simulink model "test1_v4"  (R2018a)
settings: Solver=VariableStepAuto  StartTime=0.0  StopTime=100  FixedStep=0.01  RelTol=1e-3  EnableMultiTasking=on
InitFcn:
  | run constants
values from neighbouring files (symbols this model uses):
  F_0 = [0 0 0]    [constants2.m]
  phi_noise = noise_att_on * noise_att_mag    [constants2.m]
  pm_0 = [0 0 0]    [constants2.m]
  Psi_noise = noise_att_on * noise_att_mag    [constants2.m]
  R = (RE + 700*1000)    (= 7078000)    [constants2.m]
  T_d = Td_on * [0.001 0.001 0.001]    [constants2.m]
  theta_noise = noise_att_on * noise_att_mag    [constants2.m]
  Vm_0 = [0 Vc 0]    [constants2.m]
  xme_0 = [1 2 3]    [constants2.m]
undefined symbols (not defined in the file or in its folder): Discrete, n, phi_D, phi_I, phi_P, pqr_noise, Psi_D, Psi_I, Psi_P, theta_D, theta_I, theta_P, Time
libraries: shared6dof x5, simulink x4, shared6dofsys x3, sharedutil x1, sharedTrackingLibrary x1, ctrlSharedLib x1
settings Model: PacingRate=1000  Creator=Matt  LastModifiedBy=matth
settings SolverCC: AutoInsertRateTranBlk=on
settings DataIOCC: SaveOutput=off  SaveTime=off
settings OptimizationCC: DefaultParameterBehavior=Inlined  InlineInvariantSignals=on  EnhancedBackFolding=on  PassReuseOutputArgsAs=Individual arguments  StateBitsets=on  DataBitsets=on  ZeroExternalMemoryAtStartup=off  ZeroInternalMemoryAtStartup=off  NoFixptDivByZeroProtection=on  LifeSpan=1  OptimizeBlockOrder=speed  DifferentSizesBufferReuse=on
settings DebuggingCC: ParameterTunabilityLossMsg=error
settings HardwareCC: ProdBitPerPointer=32  ProdBitPerSizeT=32  ProdBitPerPtrDiffT=32  ProdLargestAtomicFloat=None  ProdIntDivRoundTo=Floor  ProdWordSize=32  ProdHWDeviceType=Generic->Custom
settings SFSimCC: MATLABDynamicMemAlloc=off
settings RTWCC: SystemTargetFile=ert.tlc  TLCOptions=-p0  GenCodeOnly=on  TemplateMakefile=ert_default_tmf  GenerateReport=on  RTWVerbose=off  IncludeHyperlinkInReport=on  LaunchReport=on  GenerateTraceInfo=on  GenerateTraceReport=on  GenerateTraceReportSl=on  GenerateTraceReportSf=on  GenerateTraceReportEml=on
settings CodeAppCC: ForceParamTrailComments=on  IgnoreCustomStorageClasses=off  OperatorAnnotations=on  SimulinkDataObjDesc=on  SFDataObjDesc=on  CustomSymbolStrGlobalVar=rt$N$M  CustomSymbolStrType=$N$M  CustomSymbolStrFcn=$N$M$F  CustomSymbolStrMacro=$N$M  InsertBlockDesc=on
settings ERTTargetCC: TargetLangStandard=C99 (ISO)  CodeReplacementLibrary=ISO_C  GenerateSampleERTMain=on  IncludeMdlTerminateFcn=off  SuppressErrorStatus=on  SupportAbsoluteTime=off  SupportNonFinite=off  SupportComplex=off  PurelyIntegerCode=on  InlinedParameterPlacement=NonHierarchical  RootIOFormat=Structure reference  ERTCustomFileTemplate=example_file_process.tlc

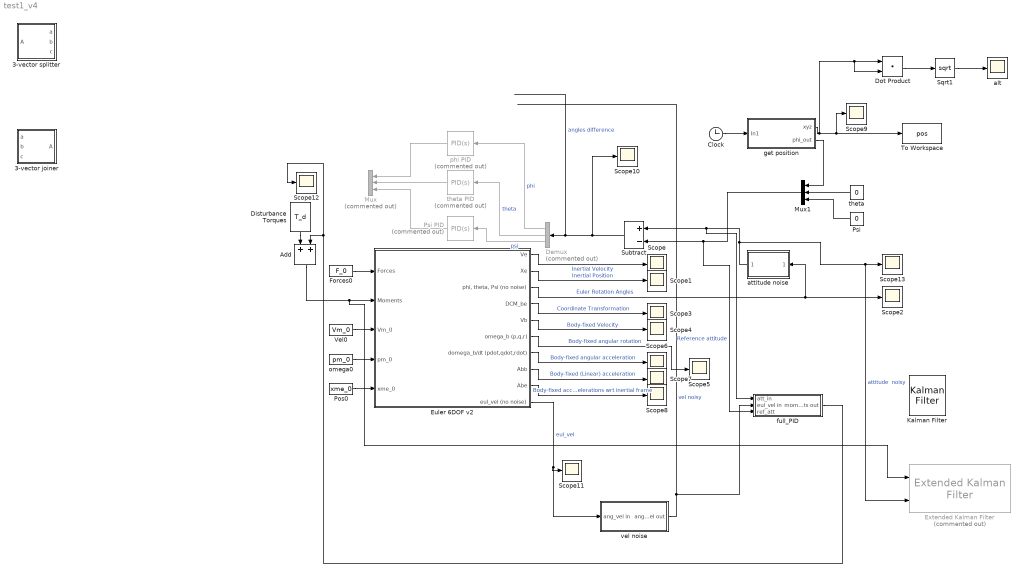
== system test1_v4 ==
  3-vector joiner : Subsystem
  3-vector splitter : Subsystem
  Add : Sum
  Clock : Clock
  Demux : Demux  Commented=on  Outputs=3
  Disturbance Torques : Constant  Value=T_d
  Dot Product : DotProduct  InputSameDT=on  OutDataTypeStr=Inherit: Inherit via internal rule
  Euler 6DOF v2 : Subsystem
  Extended Kalman Filter : sharedTrackingLibrary/Extended Kalman Filter  Commented=on  StateTransitionFcn=myStateTransitionFcn  HasStateTransitionJacobianFcn=off  HasAdditiveProcessNoise=Additive  ProcessNoise=1  HasTimeVaryingProcessNoise=off  HasStateTransitionFcnExtraArgument=1  InitialState=0  InitialStateCovariance=1  MeasurementFcn1=myMeasurementFcn  HasMeasurementJacobianFcn1=off  HasMeasurementEnablePort1=off  HasAdditiveMeasurementNoise1=Additive  MeasurementNoise1=1  HasTimeVaryingMeasurementNoise1=off  HasMeasurementFcnExtraArgument1=0  MeasurementFcn2=myMeasurementFcn  HasMeasurementJacobianFcn2=off  HasMeasurementEnablePort2=off  HasAdditiveMeasurementNoise2=Additive  MeasurementNoise2=1  HasTimeVaryingMeasurementNoise2=off  HasMeasurementFcnExtraArgument2=0  MeasurementFcn3=myMeasurementFcn  HasMeasurementJacobianFcn3=off  HasMeasurementEnablePort3=off  HasAdditiveMeasurementNoise3=Additive  MeasurementNoise3=1  HasTimeVaryingMeasurementNoise3=off  HasMeasurementFcnExtraArgument3=0  MeasurementFcn4=myMeasurementFcn  HasMeasurementJacobianFcn4=off  HasMeasurementEnablePort4=off  HasAdditiveMeasurementNoise4=Additive  MeasurementNoise4=1  HasTimeVaryingMeasurementNoise4=off  HasMeasurementFcnExtraArgument4=0  MeasurementFcn5=myMeasurementFcn  HasMeasurementJacobianFcn5=off  HasMeasurementEnablePort5=off  HasAdditiveMeasurementNoise5=Additive  MeasurementNoise5=1  HasTimeVaryingMeasurementNoise5=off  HasMeasurementFcnExtraArgument5=0  EnableMultirate=off  StateTransitionFcnSampleTime=1  MeasurementFcn1SampleTime=1  MeasurementFcn2SampleTime=1  MeasurementFcn3SampleTime=1  MeasurementFcn4SampleTime=1  MeasurementFcn5SampleTime=1  UseCurrentEstimator=off  OutputStateCovariance=off  DataType=double  SampleTime=1  NumberOfMeasurements=1
      settings: SourceProductName=Control System Toolbox  SourceProductBaseCode=CT
  Forces0 : Constant  Value=F_0
  Kalman Filter : ctrlSharedLib/Kalman Filter  TimeDomain=Discrete-Time  UseCurrentEstimator=on  ModelSource=LTI State-Space Variable  ModelSourceVariable=ss(0.95,1,1,0,1)  A=0.95  B=1  C=1  D=0  NumberOfStates=1  NumberOfInputs=1  NumberOfOutputs=1  InitialEstimateSource=Dialog  X0=0  P0=10  UseK=off  UseGH=off  NumberOfProcessNoiseInputs=1  G=1  TimeInvariantG=on  H=0  TimeInvariantH=on  Q=0.05  TimeInvariantQ=on  R=1  TimeInvariantR=on  N=0  TimeInvariantN=on  AddInputPort=on  AddEnablePort=off  OutputEstimatedY=off  OutputP=off  Ts=-1
      settings: SourceProductBaseCode=CT
  Mux : Mux  Commented=on  Inputs=3
  Mux1 : Mux  Inputs=3
  Pos0 : Constant  Value=xme_0
  "Psi " : Constant  Value=0
  Psi PID : simulink/Continuous/PID Controller  Commented=on  Controller=PID  TimeDomain=Continuous-time  SampleTime=-1  IntegratorMethod=Forward Euler  FilterMethod=Forward Euler  Form=Parallel  UseFilter=on  ControllerParametersSource=internal  P=-7886.12074600839  I=-460.070676690981  D=-30034.6975048403  N=1142.8279760416  InitialConditionSource=internal  InitialConditionForIntegrator=0  InitialConditionForFilter=0  ExternalReset=none  LimitOutput=off  UpperSaturationLimit=inf  LowerSaturationLimit=-inf  LinearizeAsGain=on  AntiWindupMode=none  Kb=1  TrackingMode=off  Kt=1  PParamMin=[]  PParamMax=[]  IParamMin=[]  IParamMax=[]  DParamMin=[]  DParamMax=[]  NParamMin=[]  NParamMax=[]  KbParamMin=[]  KbParamMax=[]  KtParamMin=[]  KtParamMax=[]  POutMin=[]  POutMax=[]  IOutMin=[]  IOutMax=[]  DOutMin=[]  DOutMax=[]  NOutMin=[]  NOutMax=[]  KbOutMin=[]  KbOutMax=[]  KtOutMin=[]  KtOutMax=[]  IntegratorOutMin=[]  IntegratorOutMax=[]  FilterOutMin=[]  FilterOutMax=[]  SumOutMin=[]  SumOutMax=[]  SumI1OutMin=[]  SumI1OutMax=[]  SumI2OutMin=[]  SumI2OutMax=[]  SumI3OutMin=[]  SumI3OutMax=[]  SumDOutMin=[]  SumDOutMax=[]  SaturationOutMin=[]  SaturationOutMax=[]  IntegratorContinuousStateAttributes=''  IntegratorStateMustResolveToSignalObject=off  IntegratorRTWStateStorageClass=Auto  FilterContinuousStateAttributes=''  FilterStateMustResolveToSignalObject=off  FilterRTWStateStorageClass=Auto  DifferentiatorICPrevScaledInput=0  DifferentiatorOutMin=[]  DifferentiatorOutMax=[]  FilterDiffOutCoefMin=[]  FilterDiffOutCoefMax=[]  SumDenOutMin=[]  SumDenOutMax=[]  SumNumOutMin=[]  SumNumOutMax=[]  ReciprocalOutMin=[]  ReciprocalOutMax=[]  DivideOutMin=[]  DivideOutMax=[]  TunerSelectOption=Transfer Function Based (PID Tuner App)
  Scope{,1..13} (14 alike) : Scope
  Sqrt1 : Sqrt  SaturateOnIntegerOverflow=on
  Subtract : Sum  Inputs=+-
  To Workspace : ToWorkspace  VariableName=pos  SaveFormat=Timeseries  SampleTime=-1
  Vel0 : Constant  Value=Vm_0
  alt : Scope
  attitude noise : Subsystem
  "full_PID " : Subsystem
  get position : Subsystem
  "omega0 " : Constant  Value=pm_0
  "phi PID " : simulink/Continuous/PID Controller  Commented=on  Controller=PID  TimeDomain=Continuous-time  SampleTime=-1  IntegratorMethod=Forward Euler  FilterMethod=Forward Euler  Form=Parallel  UseFilter=on  ControllerParametersSource=internal  P=-464.198158177747  I=-21.7313338529705  D=-2434.80245399495  N=5.45397025421619  InitialConditionSource=internal  InitialConditionForIntegrator=0  InitialConditionForFilter=0  ExternalReset=none  LimitOutput=off  UpperSaturationLimit=inf  LowerSaturationLimit=-inf  LinearizeAsGain=on  AntiWindupMode=none  Kb=1  TrackingMode=off  Kt=1  PParamMin=[]  PParamMax=[]  IParamMin=[]  IParamMax=[]  DParamMin=[]  DParamMax=[]  NParamMin=[]  NParamMax=[]  KbParamMin=[]  KbParamMax=[]  KtParamMin=[]  KtParamMax=[]  POutMin=[]  POutMax=[]  IOutMin=[]  IOutMax=[]  DOutMin=[]  DOutMax=[]  NOutMin=[]  NOutMax=[]  KbOutMin=[]  KbOutMax=[]  KtOutMin=[]  KtOutMax=[]  IntegratorOutMin=[]  IntegratorOutMax=[]  FilterOutMin=[]  FilterOutMax=[]  SumOutMin=[]  SumOutMax=[]  SumI1OutMin=[]  SumI1OutMax=[]  SumI2OutMin=[]  SumI2OutMax=[]  SumI3OutMin=[]  SumI3OutMax=[]  SumDOutMin=[]  SumDOutMax=[]  SaturationOutMin=[]  SaturationOutMax=[]  IntegratorContinuousStateAttributes=''  IntegratorStateMustResolveToSignalObject=off  IntegratorRTWStateStorageClass=Auto  FilterContinuousStateAttributes=''  FilterStateMustResolveToSignalObject=off  FilterRTWStateStorageClass=Auto  DifferentiatorICPrevScaledInput=0  DifferentiatorOutMin=[]  DifferentiatorOutMax=[]  FilterDiffOutCoefMin=[]  FilterDiffOutCoefMax=[]  SumDenOutMin=[]  SumDenOutMax=[]  SumNumOutMin=[]  SumNumOutMax=[]  ReciprocalOutMin=[]  ReciprocalOutMax=[]  DivideOutMin=[]  DivideOutMax=[]  TunerSelectOption=Transfer Function Based (PID Tuner App)
  theta : Constant  Value=0
  theta PID : simulink/Continuous/PID Controller  Commented=on  Controller=PID  TimeDomain=Continuous-time  SampleTime=-1  IntegratorMethod=Forward Euler  FilterMethod=Forward Euler  Form=Parallel  UseFilter=on  ControllerParametersSource=internal  P=-568.423410964435  I=-28.5001924417647  D=-2213.03320065217  N=10.4897155810233  InitialConditionSource=internal  InitialConditionForIntegrator=0  InitialConditionForFilter=0  ExternalReset=none  LimitOutput=off  UpperSaturationLimit=inf  LowerSaturationLimit=-inf  LinearizeAsGain=on  AntiWindupMode=none  Kb=1  TrackingMode=off  Kt=1  PParamMin=[]  PParamMax=[]  IParamMin=[]  IParamMax=[]  DParamMin=[]  DParamMax=[]  NParamMin=[]  NParamMax=[]  KbParamMin=[]  KbParamMax=[]  KtParamMin=[]  KtParamMax=[]  POutMin=[]  POutMax=[]  IOutMin=[]  IOutMax=[]  DOutMin=[]  DOutMax=[]  NOutMin=[]  NOutMax=[]  KbOutMin=[]  KbOutMax=[]  KtOutMin=[]  KtOutMax=[]  IntegratorOutMin=[]  IntegratorOutMax=[]  FilterOutMin=[]  FilterOutMax=[]  SumOutMin=[]  SumOutMax=[]  SumI1OutMin=[]  SumI1OutMax=[]  SumI2OutMin=[]  SumI2OutMax=[]  SumI3OutMin=[]  SumI3OutMax=[]  SumDOutMin=[]  SumDOutMax=[]  SaturationOutMin=[]  SaturationOutMax=[]  IntegratorContinuousStateAttributes=''  IntegratorStateMustResolveToSignalObject=off  IntegratorRTWStateStorageClass=Auto  FilterContinuousStateAttributes=''  FilterStateMustResolveToSignalObject=off  FilterRTWStateStorageClass=Auto  DifferentiatorICPrevScaledInput=0  DifferentiatorOutMin=[]  DifferentiatorOutMax=[]  FilterDiffOutCoefMin=[]  FilterDiffOutCoefMax=[]  SumDenOutMin=[]  SumDenOutMax=[]  SumNumOutMin=[]  SumNumOutMax=[]  ReciprocalOutMin=[]  ReciprocalOutMax=[]  DivideOutMin=[]  DivideOutMax=[]  TunerSelectOption=Transfer Function Based (PID Tuner App)
  "vel noise " : Subsystem
  wires:
  Euler 6DOF v2/1(Ve) -> Scope/1  "Inertial Velocity"
  Euler 6DOF v2/2(Xe) -> Scope1/1  "Inertial Position"
  Euler 6DOF v2/3("phi, theta, Psi (no noise)") -> attitude noise/1(att_in), Scope2/1  "Euler Rotation Angles"
  Euler 6DOF v2/4(DCM_be) -> Scope3/1  "Coordinate Transformation"
  Euler 6DOF v2/5(Vb) -> Scope4/1  "Body-fixed Velocity"
  Euler 6DOF v2/6(omega_b (p,q,r)) -> Scope5/1  "Body-fixed angular rotation"
  Euler 6DOF v2/7(domega_b/dt (pdot,qdot,rdot)) -> Scope6/1  "Body-fixed angular acceleration"
  Euler 6DOF v2/8(Abb) -> Scope7/1  "Body-fixed (Linear) acceleration"
  Euler 6DOF v2/9(Abe) -> Scope8/1  "Body-fixed accelerations wrt inertial frame"
  Mux1/1 -> "full_PID "/3(ref_att), Subtract/2  "Reference attitude"
  Demux/1 -> "phi PID "/1  "phi"
  Demux/2 -> theta PID/1  "theta"
  Demux/3 -> Psi PID/1  "psi"
  "phi PID "/1 -> Mux/1
  theta PID/1 -> Mux/2
  Psi PID/1 -> Mux/3
  "full_PID "/1(moments out) -> Scope12/1, Add/2
  Subtract/1 -> Scope10/1, Demux/1  "angles difference"
  Forces0/1 -> Euler 6DOF v2/1(Forces)
  Vel0/1 -> Euler 6DOF v2/3(Vm_0)
  Pos0/1 -> Euler 6DOF v2/5("xme_0 ")
  "omega0 "/1 -> Euler 6DOF v2/4("pm_0 ")
  Disturbance Torques/1 -> Add/1
  Add/1 -> Extended Kalman Filter/1, Euler 6DOF v2/2(Moments)
  Dot Product/1 -> Sqrt1/1
  Sqrt1/1 -> alt/1
  Clock/1 -> get position/1(In1)
  get position/1(xyz) -> Dot Product/2, Dot Product/1, To Workspace/1, Scope9/1
  Euler 6DOF v2/10(eul_vel (no noise)) -> "vel noise "/1(ang_vel in), Scope11/1  "eul_vel"
  attitude noise/1("att_out ") -> "full_PID "/1(att_in), Subtract/1, Extended Kalman Filter/2, Scope13/1  "attitude  noisy"
  "vel noise "/1(ang_vel out) -> "full_PID "/2(eul_vel in)  "vel noisy"
  get position/2(phi_out) -> Mux1/1
  "Psi "/1 -> Mux1/3
  theta/1 -> Mux1/2

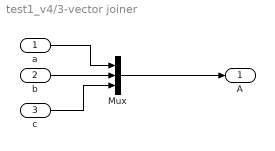
== system test1_v4/3-vector joiner ==
  a : Inport
  b : Inport  Port=2
  c : Inport  Port=3
  Mux : Mux  Inputs=3
  A : Outport
  wires:
  c/1 -> Mux/3
  a/1 -> Mux/1
  b/1 -> Mux/2
  Mux/1 -> A/1

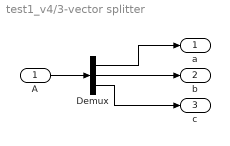
== system test1_v4/3-vector splitter ==
  A : Inport
  Demux : Demux  Outputs=3
  a : Outport
  b : Outport  Port=2
  c : Outport  Port=3
  wires:
  Demux/3 -> c/1
  Demux/2 -> b/1
  Demux/1 -> a/1
  A/1 -> Demux/1

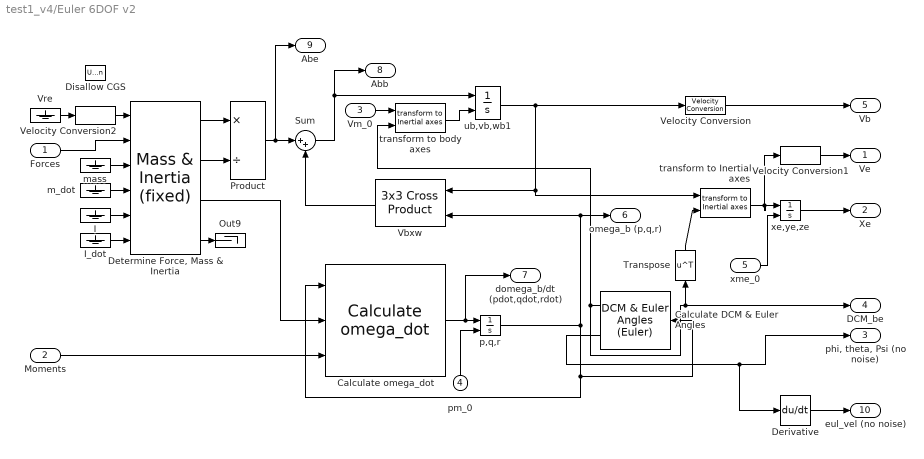
== system test1_v4/Euler 6DOF v2 ==
  Forces : Inport  Unit=N  PortDimensions=3
  Moments : Inport  Port=2  Unit=N*m  PortDimensions=3
  Vm_0 : Inport  Port=3
  "pm_0 " : Inport  Port=4
  "xme_0 " : Inport  Port=5
  Calculate DCM & Euler Angles : shared6dofsys/DCM & Euler Angles (Euler)  aMode=aMode
      settings: SourceProductName=Aerospace Blockset  SourceProductBaseCode=AE
  Calculate omega_dot : shared6dofsys/Calculate omega_dot  aMode=aMode
      settings: SourceProductName=Aerospace Blockset  SourceProductBaseCode=AE
  Derivative : Derivative
  "Determine Force, Mass & Inertia" : shared6dofsys/Mass & Inertia (fixed)  aMode=aMode
      settings: SourceProductName=Aerospace Blockset  SourceProductBaseCode=AE
  Disallow CGS : UnitConfiguration  UnitSystemsStr=English,SI,SI (extended)  AllowAllUnitSystems=off
  I : Ground
  I_dot : Ground
  Out9 : Terminator
  Product : Product  Inputs=*/  SaturateOnIntegerOverflow=on  OutDataTypeStr=Inherit: Same as first input
  Sum : Sum  Inputs=|++  SaturateOnIntegerOverflow=on
  Transpose : Math  Operator=transpose  SaturateOnIntegerOverflow=on
  Vbxw : sharedutil/3x3 Cross Product  aMode=aMode
      settings: SourceProductBaseCode=AE
  Velocity Conversion : shared6dof/6DOF (Euler Angles)/Velocity Conversion
      settings: SourceProductName=Aerospace Blockset  SourceProductBaseCode=AE
  Velocity Conversion1 : shared6dof/6DOF (Euler Angles)/Velocity Conversion1
      settings: SourceProductName=Aerospace Blockset  SourceProductBaseCode=AE
  Velocity Conversion2 : shared6dof/6DOF (Euler Angles)/Velocity Conversion2
      settings: SourceProductName=Aerospace Blockset  SourceProductBaseCode=AE
  Vre : Ground
  m_dot : Ground
  mass : Ground
  "p,q,r " : Integrator  InitialConditionSource=external  InitialCondition=pm_0
  "transform to Inertial axes " : shared6dof/6DOF (Euler Angles)/transform to Inertial axes   SystemSampleTime=-1
      settings: SourceProductName=Aerospace Blockset  SourceProductBaseCode=AE
  transform to body axes : shared6dof/6DOF (Euler Angles)/transform to Inertial axes   SystemSampleTime=-1
      settings: SourceProductName=Aerospace Blockset  SourceProductBaseCode=AE
  ub,vb,wb1 : Integrator  InitialConditionSource=external  InitialCondition=Vm_0
  xe,ye,ze : Integrator  InitialConditionSource=external  InitialCondition=xme_0
  Ve : Outport  Unit=m/s
  Xe : Outport  Port=2  Unit=m
  "phi, theta, Psi (no noise)" : Outport  Port=3  Unit=rad
  DCM_be : Outport  Port=4  Unit=1
  Vb : Outport  Port=5  Unit=m/s
  omega_b (p,q,r) : Outport  Port=6  Unit=rad/s
  domega_b/dt (pdot,qdot,rdot) : Outport  Port=7  Unit=rad/s^2
  Abb : Outport  Port=8  Unit=m/s^2
  Abe : Outport  Port=9  Unit=m/s^2
  eul_vel (no noise) : Outport  Port=10
  wires:
  Calculate DCM & Euler Angles/1 -> transform to body axes/2, Transpose/1, DCM_be/1
  Vbxw/1 -> Sum/2
  Velocity Conversion/1 -> Vb/1
  xe,ye,ze/1 -> Xe/1
  Vre/1 -> Velocity Conversion2/1
  Calculate DCM & Euler Angles/2 -> Derivative/1, "phi, theta, Psi (no noise)"/1
  "p,q,r "/1 -> Calculate omega_dot/1, Calculate DCM & Euler Angles/1, omega_b (p,q,r)/1, Vbxw/2
  Product/1 -> Sum/1, Abe/1
  Moments/1 -> Calculate omega_dot/3
  "Determine Force, Mass & Inertia"/2 -> Product/2
  "transform to Inertial axes "/1 -> xe,ye,ze/1, Velocity Conversion1/1
  "Determine Force, Mass & Inertia"/4 -> Out9/1
  Transpose/1 -> "transform to Inertial axes "/2
  mass/1 -> "Determine Force, Mass & Inertia"/3
  Velocity Conversion1/1 -> Ve/1
  Calculate omega_dot/1 -> "p,q,r "/1, domega_b/dt (pdot,qdot,rdot)/1
  I/1 -> "Determine Force, Mass & Inertia"/5
  "Determine Force, Mass & Inertia"/3 -> Calculate omega_dot/2
  ub,vb,wb1/1 -> "transform to Inertial axes "/1, Vbxw/1, Velocity Conversion/1
  "Determine Force, Mass & Inertia"/1 -> Product/1
  Forces/1 -> "Determine Force, Mass & Inertia"/2
  Velocity Conversion2/1 -> "Determine Force, Mass & Inertia"/1
  I_dot/1 -> "Determine Force, Mass & Inertia"/6
  Sum/1 -> Abb/1, ub,vb,wb1/1
  m_dot/1 -> "Determine Force, Mass & Inertia"/4
  Vm_0/1 -> transform to body axes/1
  "pm_0 "/1 -> "p,q,r "/2
  "xme_0 "/1 -> xe,ye,ze/2
  transform to body axes/1 -> ub,vb,wb1/2
  Derivative/1 -> eul_vel (no noise)/1

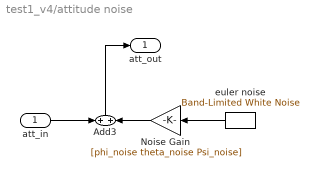
== system test1_v4/attitude noise ==
  att_in : Inport
  Add3 : Sum
  Noise Gain : Gain  Gain=[phi_noise theta_noise Psi_noise]
  euler noise : simulink/Sources/Band-Limited White Noise  Cov=[0.1]  Ts=0.1  seed=[23341]
  "att_out " : Outport
  wires:
  euler noise/1 -> Noise Gain/1
  Noise Gain/1 -> Add3/2
  att_in/1 -> Add3/1
  Add3/1 -> "att_out "/1

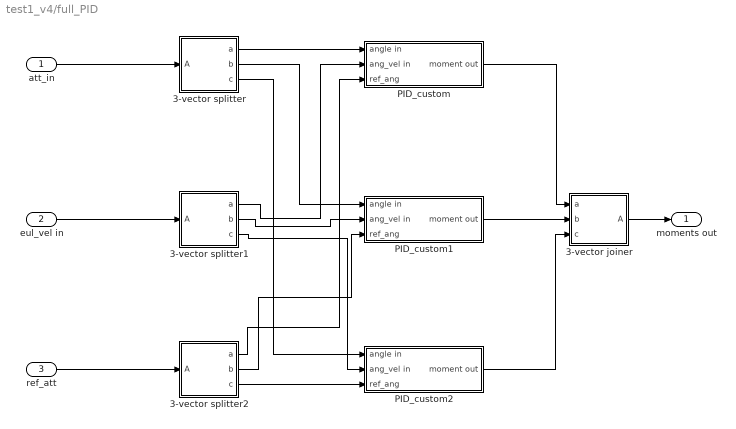
== system test1_v4/full_PID  ==
  att_in : Inport
  eul_vel in : Inport  Port=2
  ref_att : Inport  Port=3
  3-vector joiner : Subsystem
  3-vector splitter : Subsystem
  3-vector splitter1 : Subsystem
  3-vector splitter2 : Subsystem
  PID_custom : Subsystem
  PID_custom1 : Subsystem
  PID_custom2 : Subsystem
  moments out : Outport  InitialOutput=0
  wires:
  att_in/1 -> 3-vector splitter/1(A)
  eul_vel in/1 -> 3-vector splitter1/1(A)
  ref_att/1 -> 3-vector splitter2/1(A)
  3-vector splitter/1(a) -> PID_custom/1(angle in)
  3-vector splitter/2(b) -> PID_custom1/1(angle in)
  3-vector splitter/3(c) -> PID_custom2/1(angle in)
  3-vector splitter1/1(a) -> PID_custom/2(ang_vel in)
  3-vector splitter1/2(b) -> PID_custom1/2(ang_vel in)
  3-vector splitter1/3(c) -> PID_custom2/2(ang_vel in)
  3-vector splitter2/1(a) -> PID_custom/3("ref_ang ")
  3-vector splitter2/2(b) -> PID_custom1/3("ref_ang ")
  3-vector splitter2/3(c) -> PID_custom2/3("ref_ang ")
  PID_custom1/1("moment out ") -> 3-vector joiner/2(b)
  PID_custom/1("moment out ") -> 3-vector joiner/1(a)
  PID_custom2/1("moment out ") -> 3-vector joiner/3(c)
  3-vector joiner/1(A) -> moments out/1

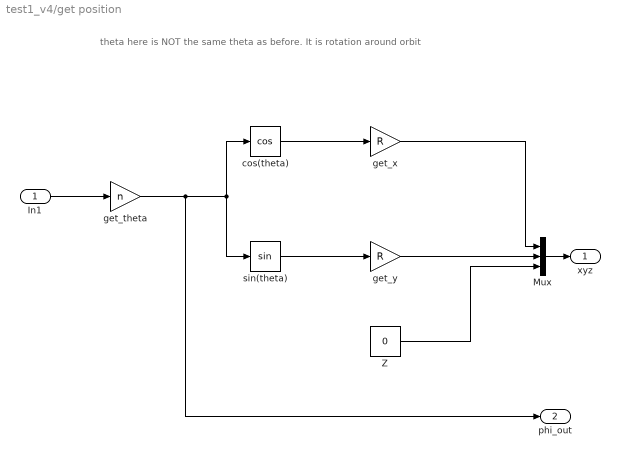
== system test1_v4/get position ==
  note: theta here is NOT the same theta as before. It is rotation around orbit
  In1 : Inport
  Mux : Mux  Inputs=3
  "Z " : Constant  Value=0
  cos(theta) : Trigonometry  Operator=cos
  get_theta : Gain  Gain=n
  "get_x " : Gain  Gain=R
  get_y : Gain  Gain=R
  sin(theta) : Trigonometry
  xyz : Outport
  phi_out : Outport  Port=2
  wires:
  In1/1 -> get_theta/1
  get_theta/1 -> phi_out/1, cos(theta)/1, sin(theta)/1
  cos(theta)/1 -> "get_x "/1
  sin(theta)/1 -> get_y/1
  "Z "/1 -> Mux/3
  get_y/1 -> Mux/2
  "get_x "/1 -> Mux/1
  Mux/1 -> xyz/1

== system test1_v4/vel noise  ==
  ang_vel in : Inport
  Add : Sum
  pqr_noise : Constant  Value=pqr_noise
  ang_vel out : Outport
  wires:
  ang_vel in/1 -> Add/2
  pqr_noise/1 -> Add/1
  Add/1 -> ang_vel out/1

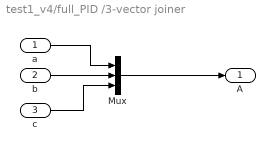
== system test1_v4/full_PID /3-vector joiner ==
  a : Inport
  b : Inport  Port=2
  c : Inport  Port=3
  Mux : Mux  Inputs=3
  A : Outport
  wires:
  c/1 -> Mux/3
  a/1 -> Mux/1
  b/1 -> Mux/2
  Mux/1 -> A/1

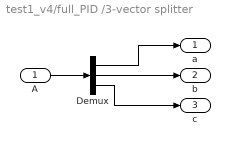
== system test1_v4/full_PID /3-vector splitter ==
  A : Inport
  Demux : Demux  Outputs=3
  a : Outport
  b : Outport  Port=2
  c : Outport  Port=3
  wires:
  Demux/3 -> c/1
  Demux/2 -> b/1
  Demux/1 -> a/1
  A/1 -> Demux/1

== system test1_v4/full_PID /3-vector splitter1 ==
  A : Inport
  Demux : Demux  Outputs=3
  a : Outport
  b : Outport  Port=2
  c : Outport  Port=3
  wires:
  Demux/3 -> c/1
  Demux/2 -> b/1
  Demux/1 -> a/1
  A/1 -> Demux/1

== system test1_v4/full_PID /3-vector splitter2 ==
  A : Inport
  Demux : Demux  Outputs=3
  a : Outport
  b : Outport  Port=2
  c : Outport  Port=3
  wires:
  Demux/3 -> c/1
  Demux/2 -> b/1
  Demux/1 -> a/1
  A/1 -> Demux/1

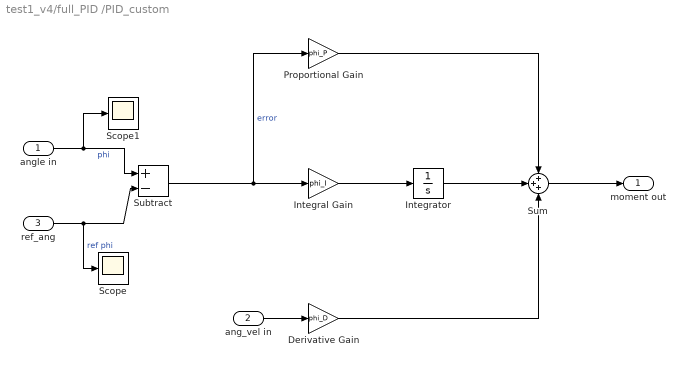
== system test1_v4/full_PID /PID_custom ==
  angle in : Inport
  ang_vel in : Inport  Port=2
  "ref_ang " : Inport  Port=3
  Derivative Gain : Gain  Gain=phi_D
  Integral Gain : Gain  Gain=phi_I
  Integrator : Integrator
  Proportional Gain : Gain  Gain=phi_P
  Scope : Scope
  Scope1 : Scope
  Subtract : Sum  Inputs=+-
  Sum : Sum  Inputs=+++
  "moment out " : Outport
  wires:
  angle in/1 -> Scope1/1, Subtract/1  "phi"
  "ref_ang "/1 -> Scope/1, Subtract/2  "ref phi"
  Subtract/1 -> Integral Gain/1, Proportional Gain/1  "error"
  Integral Gain/1 -> Integrator/1
  Proportional Gain/1 -> Sum/1
  Integrator/1 -> Sum/2
  ang_vel in/1 -> Derivative Gain/1
  Derivative Gain/1 -> Sum/3
  Sum/1 -> "moment out "/1

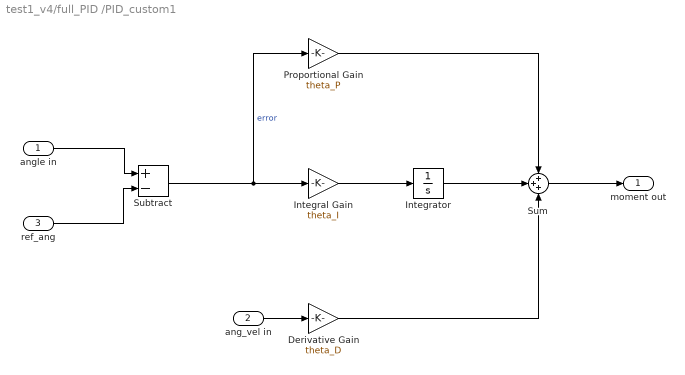
== system test1_v4/full_PID /PID_custom1 ==
  angle in : Inport
  ang_vel in : Inport  Port=2
  "ref_ang " : Inport  Port=3
  Derivative Gain : Gain  Gain=theta_D
  Integral Gain : Gain  Gain=theta_I
  Integrator : Integrator
  Proportional Gain : Gain  Gain=theta_P
  Subtract : Sum  Inputs=+-
  Sum : Sum  Inputs=+++
  "moment out " : Outport
  wires:
  angle in/1 -> Subtract/1
  "ref_ang "/1 -> Subtract/2
  Subtract/1 -> Integral Gain/1, Proportional Gain/1  "error"
  Integral Gain/1 -> Integrator/1
  Proportional Gain/1 -> Sum/1
  Integrator/1 -> Sum/2
  ang_vel in/1 -> Derivative Gain/1
  Derivative Gain/1 -> Sum/3
  Sum/1 -> "moment out "/1

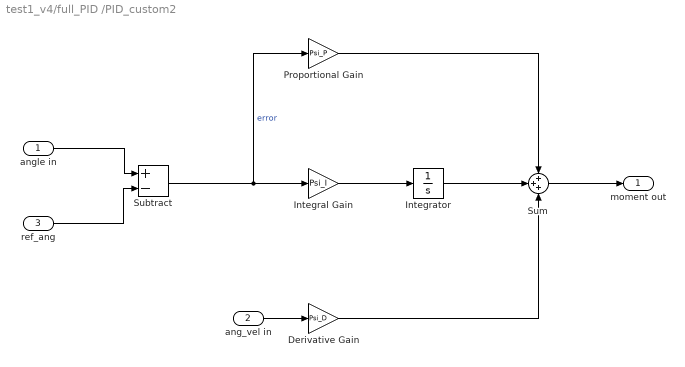
== system test1_v4/full_PID /PID_custom2 ==
  angle in : Inport
  ang_vel in : Inport  Port=2
  "ref_ang " : Inport  Port=3
  Derivative Gain : Gain  Gain=Psi_D
  Integral Gain : Gain  Gain=Psi_I
  Integrator : Integrator
  Proportional Gain : Gain  Gain=Psi_P
  Subtract : Sum  Inputs=+-
  Sum : Sum  Inputs=+++
  "moment out " : Outport
  wires:
  angle in/1 -> Subtract/1
  "ref_ang "/1 -> Subtract/2
  Subtract/1 -> Integral Gain/1, Proportional Gain/1  "error"
  Integral Gain/1 -> Integrator/1
  Proportional Gain/1 -> Sum/1
  Integrator/1 -> Sum/2
  ang_vel in/1 -> Derivative Gain/1
  Derivative Gain/1 -> Sum/3
  Sum/1 -> "moment out "/1
